simulink model "myFirstController_sim_template"  (R2019a)
settings: Solver=ode45  StartTime=0.0  StopTime=15  RelTol=1e-3  EnableMultiTasking=on
values from neighbouring files (symbols this model uses):
  A = [0.7115 -0.4345; 0.4345 0.8853]    [generateMyFirstController.m]    (also in generateMyParametricLowLevelController.m = [1.1 1; 0 1])
  B = [0.2173; 0.0573]    [generateMyFirstController.m]    (also in generateMyParametricLowLevelController.m = [1; 0.5])
  C = eye(nx)    [generateMyFirstController.m]    (also in generateMyParametricLowLevelController.m)
  D = zeros(nx,1)    [generateMyFirstController.m]    (also in generateMyParametricLowLevelController.m = zeros(nx,nu))
  x0 = zeros(model.N*model.nvar,1)    [generateMyFirstController.m]
  x_init = [0; 6]    [generateMyFirstController.m]    (also in generateMyParametricLowLevelController.m = [-4; 2])
settings Model: Creator=Juan  LastModifiedBy=UrosMarkovic
settings DataIOCC: LimitDataPoints=on  SaveFormat=Array  SignalLoggingSaveFormat=ModelDataLogs  ReturnWorkspaceOutputs=off
settings OptimizationCC: LifeSpan=inf
settings DebuggingCC: UnderspecifiedInitializationDetection=Classic  MergeDetectMultiDrivingBlocksExec=none  SolverPrmCheckMsg=warning  MultiTaskDSMMsg=warning  MultiTaskCondExecSysMsg=none  StateNameClashWarn=warning  SFUnexpectedBacktrackingDiag=warning  SFNoUnconditionalDefaultTransitionDiag=warning  SFExecutionAtInitializationDiag=none  ArithmeticOperatorsInVariantConditions=warning
settings HardwareCC: ProdBitPerPointer=32  ProdBitPerSizeT=32  ProdBitPerPtrDiffT=32  ProdLargestAtomicFloat=None  ProdIntDivRoundTo=Undefined  ProdEndianess=Unspecified  ProdWordSize=32  ProdHWDeviceType=32-bit Generic
settings ModelReferenceCC: PropagateSignalLabelsOutOfModel=off
settings SFSimCC: SimUseLocalCustomCode=off
settings RTWCC: RTWUseLocalCustomCode=off
settings CodeAppCC: StateflowObjectComments=on
settings GRTTargetCC: TargetLangStandard=C89/C90 (ANSI)  GeneratePreprocessorConditionals=Disable all
settings ConfigComp: CovMetricSettings=dw  CovHtmlReporting=on  CovSaveCumulativeToWorkspaceVar=on  CovSaveSingleToWorkspaceVar=on  CovExternalEMLEnable=off  CovSFcnEnable=off

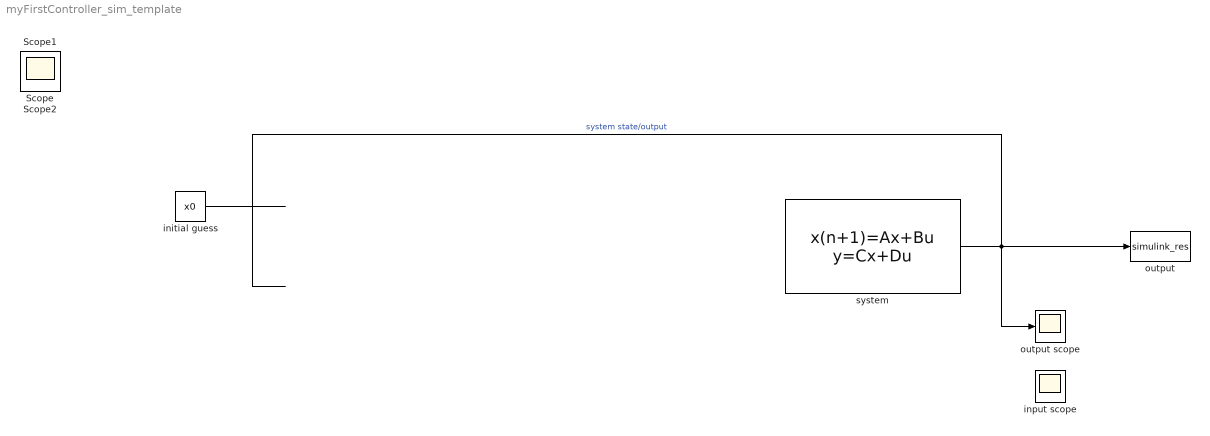
== system myFirstController_sim_template ==
  "initial guess " : Constant  Value=x0  VectorParams1D=off
  input scope : Scope
  output : ToWorkspace  VariableName=simulink_res  SaveFormat=Timeseries  SampleTime=-1
  output scope : Scope
  system : DiscreteStateSpace  A=A  B=B  C=C  D=D  InitialCondition=x_init
  Scope : Scope
  Scope1 : Scope
  Scope2 : Scope
  wires:
  system/1 -> output scope/1, output/1  "system state/output"
  ? -> input scope/1, system/1
  "initial guess "/1 -> ?
